simulink model "HW02_Tirel_Sim_Mot"  (R2020b)
settings: Solver=VariableStepAuto  StartTime=0.0  StopTime=1  RelTol=1e-3
values from neighbouring files (symbols this model uses):
  Bm = 1.02*10^-9    (= 1.02e-09)    [HW02_Tirel_Mat_Mot.m]
  Jm = 9.5*10^-10    (= 9.5e-10)    [HW02_Tirel_Mat_Mot.m]
  ke = 0.000114    [HW02_Tirel_Mat_Mot.m]
  km = 0.00109    [HW02_Tirel_Mat_Mot.m]
  La = 28*10^-6    (= 2.8e-05)    [HW02_Tirel_Mat_Mot.m]
  Ra = 8.8    [HW02_Tirel_Mat_Mot.m]
  Tl = MTl/2    (= 0.000366)    [HW02_Tirel_Mat_Mot.m]
  Ts = 0.000011    (= 1.1e-05)    [HW02_Tirel_Mat_Mot.m]
undefined symbols (not defined in the file or in its folder): K, K1
libraries: simulink x2, cstblocks x2
settings Model: Creator=DELL  LastModifiedBy=DELL

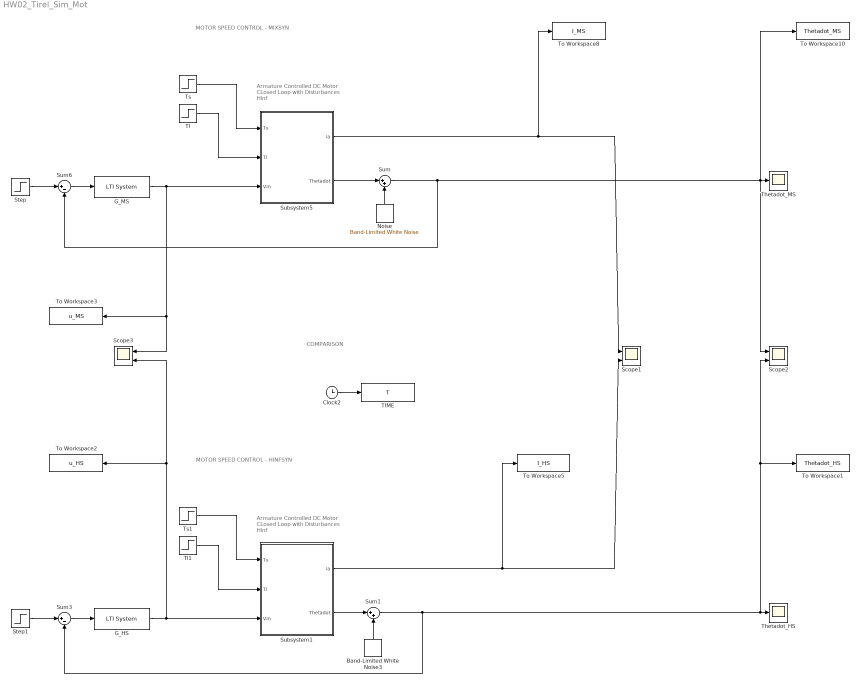
== system HW02_Tirel_Sim_Mot ==
  note: COMPARISON
  note: MOTOR SPEED CONTROL - MIXSYN
  note: Armature Controlled DC Motor
      | CLosed Loop with Disturbances Hinf
  note: Armature Controlled DC Motor
      | CLosed Loop with Disturbances Hinf
  note: MOTOR SPEED CONTROL - HINFSYN
  Band-Limited White Noise3 : simulink/Sources/Band-Limited White Noise  Cov=[0.001]  Ts=0.001  seed=[23341]
  Clock2 : Clock
  G_HS : cstblocks/LTI System  sys=tf(K1)  IC=[]
  G_MS : cstblocks/LTI System  sys=tf(K)  IC=[]
  Noise : simulink/Sources/Band-Limited White Noise  Cov=[0.001]  Ts=0.001  seed=[23341]
  Scope1 : Scope  NumInputPorts=2
  Scope2 : Scope  NumInputPorts=2
  Scope3 : Scope  NumInputPorts=2
  Step : Step  Time=0  After=25000  SampleTime=0
  Step1 : Step  Time=0  After=25000  SampleTime=0
  Subsystem1 : Subsystem
  Subsystem5 : Subsystem
  Sum : Sum  Inputs=|++
  Sum1 : Sum  Inputs=|++
  Sum3 : Sum  Inputs=|+-
  Sum6 : Sum  Inputs=|+-
  TIME : ToWorkspace  VariableName=T  SampleTime=-1
  Thetadot_HS : Scope
  Thetadot_MS : Scope
  Tl : Step  Time=0  After=Tl  SampleTime=0
  Tl1 : Step  Time=0  After=Tl  SampleTime=0
  To Workspace1 : ToWorkspace  VariableName=Thetadot_HS  SampleTime=-1
  To Workspace10 : ToWorkspace  VariableName=Thetadot_MS  SampleTime=-1
  To Workspace2 : ToWorkspace  VariableName=u_HS  SampleTime=-1
  To Workspace3 : ToWorkspace  VariableName=u_MS  SampleTime=-1
  To Workspace5 : ToWorkspace  VariableName=I_HS  SampleTime=-1
  To Workspace8 : ToWorkspace  VariableName=I_MS  SampleTime=-1
  Ts : Step  Time=0  After=Ts  SampleTime=0
  Ts1 : Step  Time=0  After=Ts  SampleTime=0
  wires:
  Tl/1 -> Subsystem5/2(Tl)
  Subsystem5/1(ia) -> Scope1/1, To Workspace8/1
  Ts/1 -> Subsystem5/1(Ts)
  Step/1 -> Sum6/1
  Sum6/1 -> G_MS/1
  G_MS/1 -> Subsystem5/3(Vm), Scope3/1, To Workspace3/1
  Tl1/1 -> Subsystem1/2(Tl)
  Subsystem1/1(ia) -> Scope1/2, To Workspace5/1
  Ts1/1 -> Subsystem1/1(Ts)
  Step1/1 -> Sum3/1
  Sum3/1 -> G_HS/1
  G_HS/1 -> To Workspace2/1, Scope3/2, Subsystem1/3(Vm)
  Subsystem5/2(Thetadot) -> Sum/1
  Sum/1 -> Sum6/2, To Workspace10/1, Thetadot_MS/1, Scope2/1
  Subsystem1/2(Thetadot) -> Sum1/1
  Sum1/1 -> Sum3/2, To Workspace1/1, Scope2/2, Thetadot_HS/1
  Clock2/1 -> TIME/1
  Noise/1 -> Sum/2
  Band-Limited White Noise3/1 -> Sum1/2

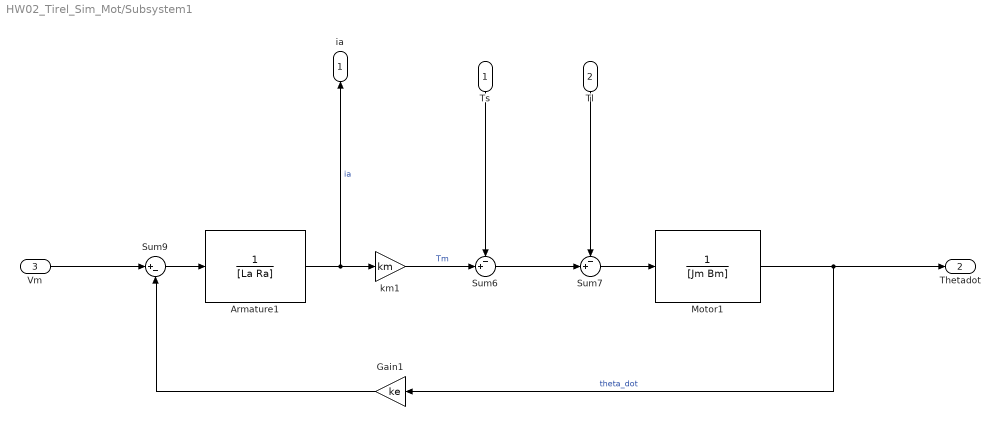
== system HW02_Tirel_Sim_Mot/Subsystem1 ==
  Ts : Inport
  Tl : Inport  Port=2
  Vm : Inport  Port=3
  Armature1 : TransferFcn  Denominator=[La Ra]
  Gain1 : Gain  Gain=ke
  Motor1 : TransferFcn  Denominator=[Jm Bm]
  Sum6 : Sum  Inputs=-+|
  Sum7 : Sum  Inputs=-+|
  Sum9 : Sum  Inputs=|+-
  km1 : Gain  Gain=km
  ia : Outport
  Thetadot : Outport  Port=2
  wires:
  Sum9/1 -> Armature1/1
  Gain1/1 -> Sum9/2
  Armature1/1 -> ia/1, km1/1  "ia"
  Motor1/1 -> Thetadot/1, Gain1/1  "theta_dot"
  Sum6/1 -> Sum7/2
  Sum7/1 -> Motor1/1
  Tl/1 -> Sum7/1
  km1/1 -> Sum6/2  "Tm"
  Vm/1 -> Sum9/1
  Ts/1 -> Sum6/1

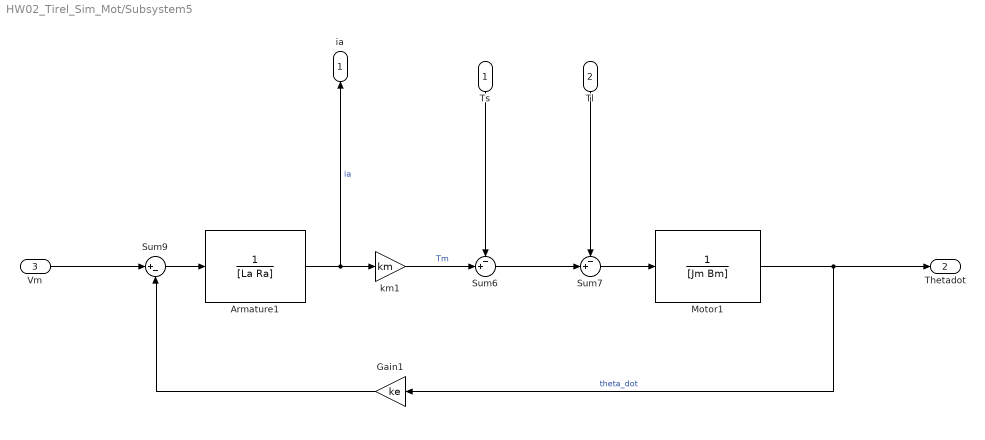
== system HW02_Tirel_Sim_Mot/Subsystem5 ==
  Ts : Inport
  Tl : Inport  Port=2
  Vm : Inport  Port=3
  Armature1 : TransferFcn  Denominator=[La Ra]
  Gain1 : Gain  Gain=ke
  Motor1 : TransferFcn  Denominator=[Jm Bm]
  Sum6 : Sum  Inputs=-+|
  Sum7 : Sum  Inputs=-+|
  Sum9 : Sum  Inputs=|+-
  km1 : Gain  Gain=km
  ia : Outport
  Thetadot : Outport  Port=2
  wires:
  Sum9/1 -> Armature1/1
  Gain1/1 -> Sum9/2
  Armature1/1 -> ia/1, km1/1  "ia"
  Motor1/1 -> Thetadot/1, Gain1/1  "theta_dot"
  Sum6/1 -> Sum7/2
  Sum7/1 -> Motor1/1
  Tl/1 -> Sum7/1
  km1/1 -> Sum6/2  "Tm"
  Vm/1 -> Sum9/1
  Ts/1 -> Sum6/1
